simulink model "MicrogridControl"  (R2025b)
settings: Solver=VariableStepAuto  StartTime=0.0  StopTime=8  FixedStep=Ts  RelTol=1e-3
PreLoadFcn:
  | NormalOperation;
  | MicrogridControlParam;
undefined symbols (not defined in the file): base, bessModeInitial, bessSystem, bessVoltage, breakerStatus, DiscIntNeverNeededParam, ee_sli_rtmsupport, event, gcbh, generator, gflInverter, gfmInverter, Inertia, lineInductance, lineResistance, machine, plannedIsland, pmsm, powerLimit, powerQuality, PV, PVInverter, ref, resync, solar, solarInsolationChange, systemFrequency, Ts, windController, windSystem, windTurbine
libraries: nesl_utility x234, ee_lib x174, fl_lib x143, eeGeneralControl x137, simulink x78, eeTransforms x47, slpidlib x23, nesl_utility_internal x12, eePwmGenerator x9, eeSinusoidalMeasurementV2 x9, custom_lib x7, batteryecm_lib x6
(part 5 of 25)

== system MicrogridControl/Subsystem/Subsystem1 ==
  Current and Voltage Sensor (Three-Phase) : ee_lib/Sensors & Transducers/Current and Voltage Sensor (Three-Phase)  vMeasurementType=ee.enum.vmeasurement.ll  outputUnit=ee.enum.unit.si  SRated=100e6 A*V  VRated=24e3 V  I_specify=off  I_priority=None  I=[0, 0, 0] A  I_nominal_specify=off  I_nominal_value=1  I_nominal_unit=A  V_specify=off  V_priority=None  V=[0, 0, 0] V  V_nominal_specify=off  V_nominal_value=1  V_nominal_unit=V
      settings: InternalSimscapePortConfiguration="{\"Bottom\":[],\"Left\":[{\"id\":\"N1\",\"label\":\"~1\",\"type\":\"foundation.electrical.three_phase\"}],\"Right\":[{\"id\":\"V_output\",\"label\":\"V\",\"type\":\"output\"},{\"id\":\"I_output\",\"label\":\"I\",\"type\":\"output\"},{\"id\":\"N2\",\"label\":\"~2\",\"type\":\"foundation.electrical.three_phase\"}],\"Top\":[]}"
  Low-Pass Filter (Discrete or Continuous) : eeGeneralControl/Low-Pass Filter (Discrete or Continuous)  K=1  T=0.1  B=inf  A=-inf  init_option=Inherited from block input  x0=0  Ts=-1
  Low-Pass Filter (Discrete or Continuous)1 : eeGeneralControl/Low-Pass Filter (Discrete or Continuous)  K=1  T=0.1  B=inf  A=-inf  init_option=Inherited from block input  x0=0  Ts=-1
  PS-Simulink Converter : nesl_utility/PS-Simulink Converter  PhysicalDomain=network_engine_domain  SubClassName=ps_output  LeftPortType=input  RightPortType=output  PseudoPeriodic=off  Frequencies=[]  VectorFormat=inherit  Unit=inherit  AffineConversion=off
  PS-Simulink Converter1 : nesl_utility/PS-Simulink Converter  PhysicalDomain=network_engine_domain  SubClassName=ps_output  LeftPortType=input  RightPortType=output  PseudoPeriodic=off  Frequencies=[]  VectorFormat=inherit  Unit=inherit  AffineConversion=off
  PS-Simulink Converter2 : nesl_utility/PS-Simulink Converter  PhysicalDomain=network_engine_domain  SubClassName=ps_output  LeftPortType=input  RightPortType=output  PseudoPeriodic=off  Frequencies=[]  VectorFormat=inherit  Unit=MW  AffineConversion=off
  PS-Simulink Converter3 : nesl_utility/PS-Simulink Converter  PhysicalDomain=network_engine_domain  SubClassName=ps_output  LeftPortType=input  RightPortType=output  PseudoPeriodic=off  Frequencies=[]  VectorFormat=inherit  Unit=MW  AffineConversion=off
  Power Sensor (Three-Phase) : ee_lib/Sensors & Transducers/Power Sensor (Three-Phase)  load_type=ee.enum.passive.type_balanced.balanced  f0=60 Hz
      settings: InternalSimscapePortConfiguration="{\"Bottom\":[],\"Left\":[{\"id\":\"N1\",\"label\":\"~1\",\"type\":\"foundation.electrical.three_phase\"}],\"Right\":[{\"id\":\"N2\",\"label\":\"~2\",\"type\":\"foundation.electrical.three_phase\"}],\"Top\":[{\"id\":\"Pm\",\"label\":\"P\",\"type\":\"output\"},{\"id\":\"Qm\",\"label\":\"Q\",\"type\":\"output\"}]}"
  Scope : Scope  NumInputPorts=2
      settings: ActiveDisplayYMinimum=-13008.240762880825  ActiveDisplayYMaximum=11933.172671563581
  In : PMIOPort  Side=Left
  Out : PMIOPort  Port=2  Side=Right
  Q : Outport
  P : Outport  Port=2
  wires:
  PS-Simulink Converter/1 -> Scope/1
  PS-Simulink Converter1/1 -> Scope/2
  PS-Simulink Converter3/1 -> Low-Pass Filter (Discrete or Continuous)1/1
  PS-Simulink Converter2/1 -> Low-Pass Filter (Discrete or Continuous)/1
  Low-Pass Filter (Discrete or Continuous)/1 -> P/1
  Low-Pass Filter (Discrete or Continuous)1/1 -> Q/1
  connections:
  PS-Simulink Converter/LConn1 -- Current and Voltage Sensor (Three-Phase)/RConn1
  Power Sensor (Three-Phase)/LConn1 -- Current and Voltage Sensor (Three-Phase)/RConn3
  Current and Voltage Sensor (Three-Phase)/LConn1 -- In/RConn1
  Power Sensor (Three-Phase)/RConn1 -- Out/RConn1
  PS-Simulink Converter1/LConn1 -- Current and Voltage Sensor (Three-Phase)/RConn2
  PS-Simulink Converter2/LConn1 -- Power Sensor (Three-Phase)/LConn2
  PS-Simulink Converter3/LConn1 -- Power Sensor (Three-Phase)/LConn3

== system MicrogridControl/Subsystem1/Circuit Breaker ==
  BRK : Inport
  Data Type Conversion : DataTypeConversion  OutDataTypeStr=double  SaturateOnIntegerOverflow=off  RndMeth=Floor
  Open Resistance : Gain  Gain=5e6
  Phase Splitter : ee_lib/Connectors & References/Phase Splitter
  Phase Splitter1 : ee_lib/Connectors & References/Phase Splitter
  Simulink-PS Converter : nesl_utility/Simulink-PS Converter  PhysicalDomain=network_engine_domain  SubClassName=ps_input  LeftPortType=input  RightPortType=output  PseudoPeriodic=off  Frequencies=[]  NoiseDistribution=none  NoiseParameters=[]  Unit=1  AffineConversion=off  FilteringAndDerivatives=provide  SimscapeFilterOrder=1  InputFilterTimeConstant=0.001  UdotUserProvided=0
  Variable Resistor : fl_lib/Electrical/Electrical Elements/Variable Resistor  Rmin=1e-3 Ohm  thermalEnable=false  thermal_mass=1 J/K  i_specify=on  i_priority=None  i=0 A  i_nominal_specify=off  i_nominal_value=1  i_nominal_unit=A  v_specify=off  v_priority=None  v=0 V  v_nominal_specify=off  v_nominal_value=1  v_nominal_unit=V  T_specify=off  T_priority=None  T=300 K  T_nominal_specify=off  T_nominal_value=1  T_nominal_unit=K
  Variable Resistor1 : fl_lib/Electrical/Electrical Elements/Variable Resistor  Rmin=1e-3 Ohm  thermalEnable=false  thermal_mass=1 J/K  i_specify=on  i_priority=None  i=0 A  i_nominal_specify=off  i_nominal_value=1  i_nominal_unit=A  v_specify=off  v_priority=None  v=0 V  v_nominal_specify=off  v_nominal_value=1  v_nominal_unit=V  T_specify=off  T_priority=None  T=300 K  T_nominal_specify=off  T_nominal_value=1  T_nominal_unit=K
  Variable Resistor2 : fl_lib/Electrical/Electrical Elements/Variable Resistor  Rmin=1e-3 Ohm  thermalEnable=false  thermal_mass=1 J/K  i_specify=on  i_priority=None  i=0 A  i_nominal_specify=off  i_nominal_value=1  i_nominal_unit=A  v_specify=off  v_priority=None  v=0 V  v_nominal_specify=off  v_nominal_value=1  v_nominal_unit=V  T_specify=off  T_priority=None  T=300 K  T_nominal_specify=off  T_nominal_value=1  T_nominal_unit=K
  In : PMIOPort  Side=Left
  ~ : PMIOPort  Port=2  Side=Right
  wires:
  Data Type Conversion/1 -> Open Resistance/1
  BRK/1 -> Data Type Conversion/1
  Open Resistance/1 -> Simulink-PS Converter/1
  connections:
  Phase Splitter1/RConn2 -- Variable Resistor1/RConn1
  Variable Resistor1/LConn2 -- Phase Splitter/RConn2
  Phase Splitter1/RConn3 -- Variable Resistor2/RConn1
  Phase Splitter/RConn1 -- Variable Resistor/LConn2
  Variable Resistor2/LConn2 -- Phase Splitter/RConn3
  Phase Splitter1/RConn1 -- Variable Resistor/RConn1
  Phase Splitter1/LConn1 -- ~/RConn1
  Variable Resistor/LConn1 -- Simulink-PS Converter/RConn1 -- Variable Resistor2/LConn1 -- Variable Resistor1/LConn1
  Phase Splitter/LConn1 -- In/RConn1

== system MicrogridControl/Subsystem1/Subsystem9 ==
  Current and Voltage Sensor (Three-Phase) : ee_lib/Sensors & Transducers/Current and Voltage Sensor (Three-Phase)  vMeasurementType=ee.enum.vmeasurement.ll  outputUnit=ee.enum.unit.si  SRated=100e6 A*V  VRated=24e3 V  I_specify=off  I_priority=None  I=[0, 0, 0] A  I_nominal_specify=off  I_nominal_value=1  I_nominal_unit=A  V_specify=off  V_priority=None  V=[0, 0, 0] V  V_nominal_specify=off  V_nominal_value=1  V_nominal_unit=V
      settings: InternalSimscapePortConfiguration="{\"Bottom\":[],\"Left\":[{\"id\":\"N1\",\"label\":\"~1\",\"type\":\"foundation.electrical.three_phase\"}],\"Right\":[{\"id\":\"V_output\",\"label\":\"V\",\"type\":\"output\"},{\"id\":\"I_output\",\"label\":\"I\",\"type\":\"output\"},{\"id\":\"N2\",\"label\":\"~2\",\"type\":\"foundation.electrical.three_phase\"}],\"Top\":[]}"
  Low-Pass Filter (Discrete or Continuous) : eeGeneralControl/Low-Pass Filter (Discrete or Continuous)  K=1  T=0.1  B=inf  A=-inf  init_option=Inherited from block input  x0=0  Ts=-1
  PS-Simulink Converter : nesl_utility/PS-Simulink Converter  PhysicalDomain=network_engine_domain  SubClassName=ps_output  LeftPortType=input  RightPortType=output  PseudoPeriodic=off  Frequencies=[]  VectorFormat=inherit  Unit=inherit  AffineConversion=off
  PS-Simulink Converter1 : nesl_utility/PS-Simulink Converter  PhysicalDomain=network_engine_domain  SubClassName=ps_output  LeftPortType=input  RightPortType=output  PseudoPeriodic=off  Frequencies=[]  VectorFormat=inherit  Unit=inherit  AffineConversion=off
  PS-Simulink Converter2 : nesl_utility/PS-Simulink Converter  PhysicalDomain=network_engine_domain  SubClassName=ps_output  LeftPortType=input  RightPortType=output  PseudoPeriodic=off  Frequencies=[]  VectorFormat=inherit  Unit=MW  AffineConversion=off
  PS-Simulink Converter3 : nesl_utility/PS-Simulink Converter  PhysicalDomain=network_engine_domain  SubClassName=ps_output  LeftPortType=input  RightPortType=output  PseudoPeriodic=off  Frequencies=[]  VectorFormat=inherit  Unit=MW  AffineConversion=off
  Power Sensor (Three-Phase) : ee_lib/Sensors & Transducers/Power Sensor (Three-Phase)  load_type=ee.enum.passive.type_balanced.balanced  f0=60 Hz
      settings: InternalSimscapePortConfiguration="{\"Bottom\":[],\"Left\":[{\"id\":\"N1\",\"label\":\"~1\",\"type\":\"foundation.electrical.three_phase\"}],\"Right\":[{\"id\":\"N2\",\"label\":\"~2\",\"type\":\"foundation.electrical.three_phase\"}],\"Top\":[{\"id\":\"Pm\",\"label\":\"P\",\"type\":\"output\"},{\"id\":\"Qm\",\"label\":\"Q\",\"type\":\"output\"}]}"
  Scope : Scope  NumInputPorts=2
      settings: ActiveDisplayYMinimum=-149653.61636  ActiveDisplayYMaximum=88760.25757
  Scope1 : Scope  NumInputPorts=2
      settings: ActiveDisplayYMinimum=-1.31777056807E+6  ActiveDisplayYMaximum=1.0009721031E+6  DataLoggingVariableName=ScopeData2
  In : PMIOPort  Side=Left
  Out : PMIOPort  Port=2  Side=Right
  Q : Outport
  P : Outport  Port=2
  wires:
  PS-Simulink Converter/1 -> Scope/1
  PS-Simulink Converter1/1 -> Scope/2
  PS-Simulink Converter3/1 -> Q/1, Scope1/2
  PS-Simulink Converter2/1 -> Low-Pass Filter (Discrete or Continuous)/1, Scope1/1
  Low-Pass Filter (Discrete or Continuous)/1 -> P/1
  connections:
  PS-Simulink Converter/LConn1 -- Current and Voltage Sensor (Three-Phase)/RConn1
  Power Sensor (Three-Phase)/LConn1 -- Current and Voltage Sensor (Three-Phase)/RConn3
  Current and Voltage Sensor (Three-Phase)/LConn1 -- In/RConn1
  Power Sensor (Three-Phase)/RConn1 -- Out/RConn1
  PS-Simulink Converter1/LConn1 -- Current and Voltage Sensor (Three-Phase)/RConn2
  PS-Simulink Converter2/LConn1 -- Power Sensor (Three-Phase)/LConn2
  PS-Simulink Converter3/LConn1 -- Power Sensor (Three-Phase)/LConn3

== system MicrogridControl/Subsystem13/Subsystem ==
  Current and Voltage Sensor (Three-Phase) : ee_lib/Sensors & Transducers/Current and Voltage Sensor (Three-Phase)  vMeasurementType=ee.enum.vmeasurement.ll  outputUnit=ee.enum.unit.si  SRated=100e6 A*V  VRated=24e3 V  I_specify=off  I_priority=None  I=[0, 0, 0] A  I_nominal_specify=off  I_nominal_value=1  I_nominal_unit=A  V_specify=off  V_priority=None  V=[0, 0, 0] V  V_nominal_specify=off  V_nominal_value=1  V_nominal_unit=V
      settings: InternalSimscapePortConfiguration="{\"Bottom\":[],\"Left\":[{\"id\":\"N1\",\"label\":\"~1\",\"type\":\"foundation.electrical.three_phase\"}],\"Right\":[{\"id\":\"V_output\",\"label\":\"V\",\"type\":\"output\"},{\"id\":\"I_output\",\"label\":\"I\",\"type\":\"output\"},{\"id\":\"N2\",\"label\":\"~2\",\"type\":\"foundation.electrical.three_phase\"}],\"Top\":[]}"
  Low-Pass Filter (Discrete or Continuous) : eeGeneralControl/Low-Pass Filter (Discrete or Continuous)  K=1  T=0.1  B=inf  A=-inf  init_option=Inherited from block input  x0=0  Ts=-1
  Low-Pass Filter (Discrete or Continuous)1 : eeGeneralControl/Low-Pass Filter (Discrete or Continuous)  K=1  T=0.1  B=inf  A=-inf  init_option=Inherited from block input  x0=0  Ts=-1
  PS-Simulink Converter : nesl_utility/PS-Simulink Converter  PhysicalDomain=network_engine_domain  SubClassName=ps_output  LeftPortType=input  RightPortType=output  PseudoPeriodic=off  Frequencies=[]  VectorFormat=inherit  Unit=inherit  AffineConversion=off
  PS-Simulink Converter1 : nesl_utility/PS-Simulink Converter  PhysicalDomain=network_engine_domain  SubClassName=ps_output  LeftPortType=input  RightPortType=output  PseudoPeriodic=off  Frequencies=[]  VectorFormat=inherit  Unit=inherit  AffineConversion=off
  PS-Simulink Converter2 : nesl_utility/PS-Simulink Converter  PhysicalDomain=network_engine_domain  SubClassName=ps_output  LeftPortType=input  RightPortType=output  PseudoPeriodic=off  Frequencies=[]  VectorFormat=inherit  Unit=MW  AffineConversion=off
  PS-Simulink Converter3 : nesl_utility/PS-Simulink Converter  PhysicalDomain=network_engine_domain  SubClassName=ps_output  LeftPortType=input  RightPortType=output  PseudoPeriodic=off  Frequencies=[]  VectorFormat=inherit  Unit=MW  AffineConversion=off
  Power Sensor (Three-Phase) : ee_lib/Sensors & Transducers/Power Sensor (Three-Phase)  load_type=ee.enum.passive.type_balanced.balanced  f0=60 Hz
      settings: InternalSimscapePortConfiguration="{\"Bottom\":[],\"Left\":[{\"id\":\"N1\",\"label\":\"~1\",\"type\":\"foundation.electrical.three_phase\"}],\"Right\":[{\"id\":\"N2\",\"label\":\"~2\",\"type\":\"foundation.electrical.three_phase\"}],\"Top\":[{\"id\":\"Pm\",\"label\":\"P\",\"type\":\"output\"},{\"id\":\"Qm\",\"label\":\"Q\",\"type\":\"output\"}]}"
  Scope : Scope  NumInputPorts=2
      settings: ActiveDisplayYMinimum=-149653.61636  ActiveDisplayYMaximum=88760.25757
  In : PMIOPort  Side=Left
  Out : PMIOPort  Port=2  Side=Right
  Q : Outport
  P : Outport  Port=2
  wires:
  PS-Simulink Converter/1 -> Scope/1
  PS-Simulink Converter1/1 -> Scope/2
  PS-Simulink Converter3/1 -> Low-Pass Filter (Discrete or Continuous)1/1
  PS-Simulink Converter2/1 -> Low-Pass Filter (Discrete or Continuous)/1
  Low-Pass Filter (Discrete or Continuous)/1 -> P/1
  Low-Pass Filter (Discrete or Continuous)1/1 -> Q/1
  connections:
  PS-Simulink Converter/LConn1 -- Current and Voltage Sensor (Three-Phase)/RConn1
  Power Sensor (Three-Phase)/LConn1 -- Current and Voltage Sensor (Three-Phase)/RConn3
  Current and Voltage Sensor (Three-Phase)/LConn1 -- In/RConn1
  Power Sensor (Three-Phase)/RConn1 -- Out/RConn1
  PS-Simulink Converter1/LConn1 -- Current and Voltage Sensor (Three-Phase)/RConn2
  PS-Simulink Converter2/LConn1 -- Power Sensor (Three-Phase)/LConn2
  PS-Simulink Converter3/LConn1 -- Power Sensor (Three-Phase)/LConn3

== system MicrogridControl/Subsystem15/Circuit Breaker ==
  BRK : Inport
  Data Type Conversion : DataTypeConversion  OutDataTypeStr=double  SaturateOnIntegerOverflow=off  RndMeth=Floor
  Open Resistance : Gain  Gain=5e6
  Phase Splitter : ee_lib/Connectors & References/Phase Splitter
  Phase Splitter1 : ee_lib/Connectors & References/Phase Splitter
  Simulink-PS Converter : nesl_utility/Simulink-PS Converter  PhysicalDomain=network_engine_domain  SubClassName=ps_input  LeftPortType=input  RightPortType=output  PseudoPeriodic=off  Frequencies=[]  NoiseDistribution=none  NoiseParameters=[]  Unit=1  AffineConversion=off  FilteringAndDerivatives=provide  SimscapeFilterOrder=1  InputFilterTimeConstant=0.001  UdotUserProvided=0
  Variable Resistor : fl_lib/Electrical/Electrical Elements/Variable Resistor  Rmin=1e-3 Ohm  thermalEnable=false  thermal_mass=1 J/K  i_specify=on  i_priority=None  i=0 A  i_nominal_specify=off  i_nominal_value=1  i_nominal_unit=A  v_specify=off  v_priority=None  v=0 V  v_nominal_specify=off  v_nominal_value=1  v_nominal_unit=V  T_specify=off  T_priority=None  T=300 K  T_nominal_specify=off  T_nominal_value=1  T_nominal_unit=K
  Variable Resistor1 : fl_lib/Electrical/Electrical Elements/Variable Resistor  Rmin=1e-3 Ohm  thermalEnable=false  thermal_mass=1 J/K  i_specify=on  i_priority=None  i=0 A  i_nominal_specify=off  i_nominal_value=1  i_nominal_unit=A  v_specify=off  v_priority=None  v=0 V  v_nominal_specify=off  v_nominal_value=1  v_nominal_unit=V  T_specify=off  T_priority=None  T=300 K  T_nominal_specify=off  T_nominal_value=1  T_nominal_unit=K
  Variable Resistor2 : fl_lib/Electrical/Electrical Elements/Variable Resistor  Rmin=1e-3 Ohm  thermalEnable=false  thermal_mass=1 J/K  i_specify=on  i_priority=None  i=0 A  i_nominal_specify=off  i_nominal_value=1  i_nominal_unit=A  v_specify=off  v_priority=None  v=0 V  v_nominal_specify=off  v_nominal_value=1  v_nominal_unit=V  T_specify=off  T_priority=None  T=300 K  T_nominal_specify=off  T_nominal_value=1  T_nominal_unit=K
  In : PMIOPort  Side=Left
  ~ : PMIOPort  Port=2  Side=Right
  wires:
  Data Type Conversion/1 -> Open Resistance/1
  BRK/1 -> Data Type Conversion/1
  Open Resistance/1 -> Simulink-PS Converter/1
  connections:
  Phase Splitter1/RConn2 -- Variable Resistor1/RConn1
  Variable Resistor1/LConn2 -- Phase Splitter/RConn2
  Phase Splitter1/RConn3 -- Variable Resistor2/RConn1
  Phase Splitter/RConn1 -- Variable Resistor/LConn2
  Variable Resistor2/LConn2 -- Phase Splitter/RConn3
  Phase Splitter1/RConn1 -- Variable Resistor/RConn1
  Phase Splitter1/LConn1 -- ~/RConn1
  Variable Resistor/LConn1 -- Simulink-PS Converter/RConn1 -- Variable Resistor2/LConn1 -- Variable Resistor1/LConn1
  Phase Splitter/LConn1 -- In/RConn1

== system MicrogridControl/Subsystem15/Subsystem4 ==
  Current and Voltage Sensor (Three-Phase) : ee_lib/Sensors & Transducers/Current and Voltage Sensor (Three-Phase)  vMeasurementType=ee.enum.vmeasurement.ll  outputUnit=ee.enum.unit.si  SRated=100e6 A*V  VRated=24e3 V  I_specify=off  I_priority=None  I=[0, 0, 0] A  I_nominal_specify=off  I_nominal_value=1  I_nominal_unit=A  V_specify=off  V_priority=None  V=[0, 0, 0] V  V_nominal_specify=off  V_nominal_value=1  V_nominal_unit=V
      settings: InternalSimscapePortConfiguration="{\"Bottom\":[],\"Left\":[{\"id\":\"N1\",\"label\":\"~1\",\"type\":\"foundation.electrical.three_phase\"}],\"Right\":[{\"id\":\"V_output\",\"label\":\"V\",\"type\":\"output\"},{\"id\":\"I_output\",\"label\":\"I\",\"type\":\"output\"},{\"id\":\"N2\",\"label\":\"~2\",\"type\":\"foundation.electrical.three_phase\"}],\"Top\":[]}"
  Gain : Gain  Gain=0.5
  Low-Pass Filter (Discrete or Continuous) : eeGeneralControl/Low-Pass Filter (Discrete or Continuous)  K=1  T=0.1  B=inf  A=-inf  init_option=Inherited from block input  x0=0  Ts=-1
  Low-Pass Filter (Discrete or Continuous)1 : eeGeneralControl/Low-Pass Filter (Discrete or Continuous)  K=1  T=0.1  B=inf  A=-inf  init_option=Inherited from block input  x0=0  Ts=-1
  PS-Simulink Converter : nesl_utility/PS-Simulink Converter  PhysicalDomain=network_engine_domain  SubClassName=ps_output  LeftPortType=input  RightPortType=output  PseudoPeriodic=off  Frequencies=[]  VectorFormat=inherit  Unit=inherit  AffineConversion=off
  PS-Simulink Converter1 : nesl_utility/PS-Simulink Converter  PhysicalDomain=network_engine_domain  SubClassName=ps_output  LeftPortType=input  RightPortType=output  PseudoPeriodic=off  Frequencies=[]  VectorFormat=inherit  Unit=inherit  AffineConversion=off
  PS-Simulink Converter2 : nesl_utility/PS-Simulink Converter  PhysicalDomain=network_engine_domain  SubClassName=ps_output  LeftPortType=input  RightPortType=output  PseudoPeriodic=off  Frequencies=[]  VectorFormat=inherit  Unit=MW  AffineConversion=off
  PS-Simulink Converter3 : nesl_utility/PS-Simulink Converter  PhysicalDomain=network_engine_domain  SubClassName=ps_output  LeftPortType=input  RightPortType=output  PseudoPeriodic=off  Frequencies=[]  VectorFormat=inherit  Unit=MW  AffineConversion=off
  Power Sensor (Three-Phase) : ee_lib/Sensors & Transducers/Power Sensor (Three-Phase)  load_type=ee.enum.passive.type_balanced.balanced  f0=60 Hz
      settings: InternalSimscapePortConfiguration="{\"Bottom\":[],\"Left\":[{\"id\":\"N1\",\"label\":\"~1\",\"type\":\"foundation.electrical.three_phase\"}],\"Right\":[{\"id\":\"N2\",\"label\":\"~2\",\"type\":\"foundation.electrical.three_phase\"}],\"Top\":[{\"id\":\"Pm\",\"label\":\"P\",\"type\":\"output\"},{\"id\":\"Qm\",\"label\":\"Q\",\"type\":\"output\"}]}"
  Scope : Scope  NumInputPorts=2
      settings: ActiveDisplayYMinimum=-149653.61636  ActiveDisplayYMaximum=88760.25757
  In : PMIOPort  Side=Left
  Out : PMIOPort  Port=2  Side=Right
  Q : Outport
  P : Outport  Port=2
  wires:
  PS-Simulink Converter/1 -> Scope/1
  PS-Simulink Converter1/1 -> Scope/2
  PS-Simulink Converter2/1 -> Low-Pass Filter (Discrete or Continuous)/1
  Low-Pass Filter (Discrete or Continuous)/1 -> P/1
  PS-Simulink Converter3/1 -> Low-Pass Filter (Discrete or Continuous)1/1
  Low-Pass Filter (Discrete or Continuous)1/1 -> Q/1
  connections:
  PS-Simulink Converter/LConn1 -- Current and Voltage Sensor (Three-Phase)/RConn1
  Power Sensor (Three-Phase)/LConn1 -- Current and Voltage Sensor (Three-Phase)/RConn3
  Current and Voltage Sensor (Three-Phase)/LConn1 -- In/RConn1
  Power Sensor (Three-Phase)/RConn1 -- Out/RConn1
  PS-Simulink Converter1/LConn1 -- Current and Voltage Sensor (Three-Phase)/RConn2
  PS-Simulink Converter2/LConn1 -- Power Sensor (Three-Phase)/LConn2
  PS-Simulink Converter3/LConn1 -- Power Sensor (Three-Phase)/LConn3

== system MicrogridControl/Subsystem15/Transformer ==
  Detailed : Subsystem  VariantControl=Detailed
  Simplified : Subsystem  VariantControl=Simplified  mask{windingRatio=13500/6600}
      mask prompts: windingRatio "Winding ratio"
      mask DialogControl Container4 Prompt: General
  In : PMIOPort  Side=Left
  Out : PMIOPort  Port=2  Side=Right

== system MicrogridControl/Subsystem3/Subsystem2 ==
  Current and Voltage Sensor (Three-Phase) : ee_lib/Sensors & Transducers/Current and Voltage Sensor (Three-Phase)  vMeasurementType=ee.enum.vmeasurement.ll  outputUnit=ee.enum.unit.pu  SRated=10.5e6 A*V  VRated=11000 V  I_specify=off  I_priority=None  I=[0, 0, 0] A  I_nominal_specify=off  I_nominal_value=1  I_nominal_unit=A  V_specify=off  V_priority=None  V=[0, 0, 0] V  V_nominal_specify=off  V_nominal_value=1  V_nominal_unit=V
      settings: InternalSimscapePortConfiguration="{\"Bottom\":[],\"Left\":[{\"id\":\"N1\",\"label\":\"~1\",\"type\":\"foundation.electrical.three_phase\"}],\"Right\":[{\"id\":\"V_output\",\"label\":\"V\",\"type\":\"output\"},{\"id\":\"I_output\",\"label\":\"I\",\"type\":\"output\"},{\"id\":\"N2\",\"label\":\"~2\",\"type\":\"foundation.electrical.three_phase\"}],\"Top\":[]}"
  Low-Pass Filter (Discrete or Continuous) : eeGeneralControl/Low-Pass Filter (Discrete or Continuous)  K=1  T=0.1  B=inf  A=-inf  init_option=Inherited from block input  x0=0  Ts=-1
  Low-Pass Filter (Discrete or Continuous)1 : eeGeneralControl/Low-Pass Filter (Discrete or Continuous)  K=1  T=0.1  B=inf  A=-inf  init_option=Inherited from block input  x0=0  Ts=-1
  Low-Pass Filter (Discrete or Continuous)2 : eeGeneralControl/Low-Pass Filter (Discrete or Continuous)  K=1  T=0.001  B=inf  A=-inf  init_option=Inherited from block input  x0=0  Ts=-1
  Low-Pass Filter (Discrete or Continuous)3 : eeGeneralControl/Low-Pass Filter (Discrete or Continuous)  K=1  T=0.001  B=inf  A=-inf  init_option=Inherited from block input  x0=0  Ts=-1
  PS-Simulink Converter : nesl_utility/PS-Simulink Converter  PhysicalDomain=network_engine_domain  SubClassName=ps_output  LeftPortType=input  RightPortType=output  PseudoPeriodic=off  Frequencies=[]  VectorFormat=inherit  Unit=inherit  AffineConversion=off
  PS-Simulink Converter1 : nesl_utility/PS-Simulink Converter  PhysicalDomain=network_engine_domain  SubClassName=ps_output  LeftPortType=input  RightPortType=output  PseudoPeriodic=off  Frequencies=[]  VectorFormat=inherit  Unit=inherit  AffineConversion=off
  PS-Simulink Converter2 : nesl_utility/PS-Simulink Converter  PhysicalDomain=network_engine_domain  SubClassName=ps_output  LeftPortType=input  RightPortType=output  PseudoPeriodic=off  Frequencies=[]  VectorFormat=inherit  Unit=MW  AffineConversion=off
  PS-Simulink Converter3 : nesl_utility/PS-Simulink Converter  PhysicalDomain=network_engine_domain  SubClassName=ps_output  LeftPortType=input  RightPortType=output  PseudoPeriodic=off  Frequencies=[]  VectorFormat=inherit  Unit=MW  AffineConversion=off
  Power Sensor (Three-Phase) : ee_lib/Sensors & Transducers/Power Sensor (Three-Phase)  load_type=ee.enum.passive.type_balanced.balanced  f0=60 Hz
      settings: InternalSimscapePortConfiguration="{\"Bottom\":[],\"Left\":[{\"id\":\"N1\",\"label\":\"~1\",\"type\":\"foundation.electrical.three_phase\"}],\"Right\":[{\"id\":\"N2\",\"label\":\"~2\",\"type\":\"foundation.electrical.three_phase\"}],\"Top\":[{\"id\":\"Pm\",\"label\":\"P\",\"type\":\"output\"},{\"id\":\"Qm\",\"label\":\"Q\",\"type\":\"output\"}]}"
  Terminator : Terminator
  Terminator1 : Terminator
  In : PMIOPort  Side=Left
  Out : PMIOPort  Port=2  Side=Right
  P : Outport
  Q : Outport  Port=2
  wires:
  PS-Simulink Converter3/1 -> Low-Pass Filter (Discrete or Continuous)1/1
  PS-Simulink Converter2/1 -> Low-Pass Filter (Discrete or Continuous)/1
  Low-Pass Filter (Discrete or Continuous)/1 -> P/1
  Low-Pass Filter (Discrete or Continuous)1/1 -> Q/1
  PS-Simulink Converter/1 -> Low-Pass Filter (Discrete or Continuous)2/1
  Low-Pass Filter (Discrete or Continuous)2/1 -> Terminator/1
  PS-Simulink Converter1/1 -> Low-Pass Filter (Discrete or Continuous)3/1
  Low-Pass Filter (Discrete or Continuous)3/1 -> Terminator1/1
  connections:
  PS-Simulink Converter/LConn1 -- Current and Voltage Sensor (Three-Phase)/RConn1
  Power Sensor (Three-Phase)/LConn1 -- Current and Voltage Sensor (Three-Phase)/RConn3
  Current and Voltage Sensor (Three-Phase)/LConn1 -- In/RConn1
  Power Sensor (Three-Phase)/RConn1 -- Out/RConn1
  PS-Simulink Converter1/LConn1 -- Current and Voltage Sensor (Three-Phase)/RConn2
  PS-Simulink Converter2/LConn1 -- Power Sensor (Three-Phase)/LConn2
  PS-Simulink Converter3/LConn1 -- Power Sensor (Three-Phase)/LConn3

== system MicrogridControl/Subsystem4/Subsystem3 ==
  Current and Voltage Sensor (Three-Phase) : ee_lib/Sensors & Transducers/Current and Voltage Sensor (Three-Phase)  vMeasurementType=ee.enum.vmeasurement.ll  outputUnit=ee.enum.unit.si  SRated=100e6 A*V  VRated=24e3 V  I_specify=off  I_priority=None  I=[0, 0, 0] A  I_nominal_specify=off  I_nominal_value=1  I_nominal_unit=A  V_specify=off  V_priority=None  V=[0, 0, 0] V  V_nominal_specify=off  V_nominal_value=1  V_nominal_unit=V
      settings: InternalSimscapePortConfiguration="{\"Bottom\":[],\"Left\":[{\"id\":\"N1\",\"label\":\"~1\",\"type\":\"foundation.electrical.three_phase\"}],\"Right\":[{\"id\":\"V_output\",\"label\":\"V\",\"type\":\"output\"},{\"id\":\"I_output\",\"label\":\"I\",\"type\":\"output\"},{\"id\":\"N2\",\"label\":\"~2\",\"type\":\"foundation.electrical.three_phase\"}],\"Top\":[]}"
  Low-Pass Filter (Discrete or Continuous) : eeGeneralControl/Low-Pass Filter (Discrete or Continuous)  K=1  T=0.1  B=inf  A=-inf  init_option=Inherited from block input  x0=0  Ts=-1
  Low-Pass Filter (Discrete or Continuous)1 : eeGeneralControl/Low-Pass Filter (Discrete or Continuous)  K=1  T=0.1  B=inf  A=-inf  init_option=Inherited from block input  x0=0  Ts=-1
  PS-Simulink Converter : nesl_utility/PS-Simulink Converter  PhysicalDomain=network_engine_domain  SubClassName=ps_output  LeftPortType=input  RightPortType=output  PseudoPeriodic=off  Frequencies=[]  VectorFormat=inherit  Unit=inherit  AffineConversion=off
  PS-Simulink Converter1 : nesl_utility/PS-Simulink Converter  PhysicalDomain=network_engine_domain  SubClassName=ps_output  LeftPortType=input  RightPortType=output  PseudoPeriodic=off  Frequencies=[]  VectorFormat=inherit  Unit=inherit  AffineConversion=off
  PS-Simulink Converter2 : nesl_utility/PS-Simulink Converter  PhysicalDomain=network_engine_domain  SubClassName=ps_output  LeftPortType=input  RightPortType=output  PseudoPeriodic=off  Frequencies=[]  VectorFormat=inherit  Unit=MW  AffineConversion=off
  PS-Simulink Converter3 : nesl_utility/PS-Simulink Converter  PhysicalDomain=network_engine_domain  SubClassName=ps_output  LeftPortType=input  RightPortType=output  PseudoPeriodic=off  Frequencies=[]  VectorFormat=inherit  Unit=MW  AffineConversion=off
  Power Sensor (Three-Phase) : ee_lib/Sensors & Transducers/Power Sensor (Three-Phase)  load_type=ee.enum.passive.type_balanced.balanced  f0=60 Hz
      settings: InternalSimscapePortConfiguration="{\"Bottom\":[],\"Left\":[{\"id\":\"N1\",\"label\":\"~1\",\"type\":\"foundation.electrical.three_phase\"}],\"Right\":[{\"id\":\"N2\",\"label\":\"~2\",\"type\":\"foundation.electrical.three_phase\"}],\"Top\":[{\"id\":\"Pm\",\"label\":\"P\",\"type\":\"output\"},{\"id\":\"Qm\",\"label\":\"Q\",\"type\":\"output\"}]}"
  Scope : Scope  NumInputPorts=2
      settings: ActiveDisplayYMinimum=-149653.61636  ActiveDisplayYMaximum=88760.25757
  In : PMIOPort  Side=Left
  Out : PMIOPort  Port=2  Side=Right
  Q : Outport
  P : Outport  Port=2
  wires:
  PS-Simulink Converter/1 -> Scope/1
  PS-Simulink Converter1/1 -> Scope/2
  PS-Simulink Converter3/1 -> Low-Pass Filter (Discrete or Continuous)1/1
  PS-Simulink Converter2/1 -> Low-Pass Filter (Discrete or Continuous)/1
  Low-Pass Filter (Discrete or Continuous)/1 -> P/1
  Low-Pass Filter (Discrete or Continuous)1/1 -> Q/1
  connections:
  PS-Simulink Converter/LConn1 -- Current and Voltage Sensor (Three-Phase)/RConn1
  Power Sensor (Three-Phase)/LConn1 -- Current and Voltage Sensor (Three-Phase)/RConn3
  Current and Voltage Sensor (Three-Phase)/LConn1 -- In/RConn1
  Power Sensor (Three-Phase)/RConn1 -- Out/RConn1
  PS-Simulink Converter1/LConn1 -- Current and Voltage Sensor (Three-Phase)/RConn2
  PS-Simulink Converter2/LConn1 -- Power Sensor (Three-Phase)/LConn2
  PS-Simulink Converter3/LConn1 -- Power Sensor (Three-Phase)/LConn3

== system MicrogridControl/Wind Farm/Transformer ==
  Detailed : Subsystem  VariantControl=Detailed
  Simplified : Subsystem  VariantControl=Simplified  mask{windingRatio=690/6600}
      mask prompts: windingRatio "Winding ratio"
      mask DialogControl Container4 Prompt: General
  In : PMIOPort  Side=Left
  Out : PMIOPort  Port=2  Side=Right

== system MicrogridControl/Wind Farm/Transformer1 ==
  Detailed : Subsystem  VariantControl=Detailed
  Simplified : Subsystem  VariantControl=Simplified  mask{windingRatio=690/6600}
      mask prompts: windingRatio "Winding ratio"
      mask DialogControl Container4 Prompt: General
  In : PMIOPort  Side=Left
  Out : PMIOPort  Port=2  Side=Right

== system MicrogridControl/Wind Farm/Wind Plant Integrated ==
  LVRT : Inport
  QRef : Inport  Port=2
  WindSpeed : Inport  Port=3
  Detailed : Subsystem  VariantControl=Detailed
      settings: CopyFcn=set_param(gcbh,'LinkStatus','none');
  Simplified : Subsystem  VariantControl=Simplified
  ~ : PMIOPort  Side=Right
  Meas : Outport

== system MicrogridControl/Wind Farm/Wind Plant Integrated1 ==
  LVRT : Inport
  QRef : Inport  Port=2
  WindSpeed : Inport  Port=3
  Detailed : Subsystem  VariantControl=Detailed
      settings: CopyFcn=set_param(gcbh,'LinkStatus','none');
  Simplified : Subsystem  VariantControl=Simplified
  ~ : PMIOPort  Side=Right
  Meas : Outport

== system MicrogridControl/BESS/BESS Integrated/Detailed ==
  note: Plant
  note: Controller
  VRef : Inport
  FRef : Inport  Port=2
  PRef : Inport  Port=3
  QRef : Inport  Port=4
  Mode : Inport  Port=5
  Reset : Inport  Port=6
  BESS Controller : Subsystem  Variant=on  VariantControlMode=label  LabelModeActiveChoice=Grid Forming
  BESS Plant : Subsystem  mask(BESS Plant){converterFidelity=Average, fSw=fSw, ratedVoltage=Vac}
      mask prompts: converterFidelity "Converter Fidelity"; fSw "Switching Frequency (kHz)"; ratedVoltage "Rated voltage on AC side (V)"
      mask help: This block represents the physical interface between the battery and the power converter. It models the electrical and dynamic characteristics of the battery system connected to a converter, while expecting an external control signal for operation
      settings: CopyFcn=set_param(gcbh,'LinkStatus','none');
      mask TypeOptions converterFidelity: Converter/converterFidelity
      mask Callback converterFidelity: component.mask.converterFidelityPlant;
      mask TypeOptions fSw: Converter/fSw
      mask DialogControl Container4 Prompt: General
      mask DialogControl editBattery Prompt: Edit battery parameters
      mask DialogControl editBattery Callback:
      | blockPath = [gcb,'/','Battery'];
      | component.mask.openBlock(blockPath);
      mask DialogControl editConverter Prompt: Edit converter parameters
      mask DialogControl editConverter Callback:
      | converterFidelity = get_param(gcb,'converterFidelity');
      | blockPath = [gcb,'/','Converter','/',converterFidelity,'/','Converter'];
      | component.mask.openBlock(blockPath);
      mask Display: image('battery.png');
  Filter & Measurements : Subsystem
  ~ : PMIOPort  Side=Right
  Meas : Outport
  wires:
  BESS Plant/1(SOC) -> Filter & Measurements/1(SOC)
  FRef/1 -> BESS Controller/2(FRef)
  Mode/1 -> BESS Controller/5(Mode)
  PRef/1 -> BESS Controller/3(PRef)
  Filter & Measurements/1(VIBus) -> BESS Controller/7(VIBus)
  QRef/1 -> BESS Controller/4(QRef)
  VRef/1 -> BESS Controller/1(VRef)
  Reset/1 -> BESS Controller/6(Reset)
  Filter & Measurements/2(Meas) -> Meas/1
  BESS Controller/1(mabc) -> BESS Plant/1(mabc)
  connections:
  Filter & Measurements/RConn1 -- ~/RConn1
  BESS Plant/RConn1 -- Filter & Measurements/LConn1

== system MicrogridControl/BESS/BESS Integrated/Simplified ==
  VRef : Inport
  FRef : Inport  Port=2
  PRef : Inport  Port=3
  QRef : Inport  Port=4
  Mode : Inport  Port=5
  Reset : Inport  Port=6
  Grid Following : Subsystem  VariantControl=Grid Following  mask(BESS GFL Simplified){plantRating=plantRating, Vac=Vac, frequency=frequency, iMaxPU=iMaxPU, efficiency=efficiency, bessVoltage=baseVoltageDC, maxSOC=maxSOC, minSOC=minSOC}
      mask prompts: plantRating "BESS Rating (kW)"; Vac "Rated AC side voltage (phase-phase RMS) (V)"; frequency "Rated electrical frequency at AC side (Hz)"; iMaxPU "Maximum converter current (pu)"; efficiency "Converter Efficiency (%)"; bessVoltage "Nominal BESS voltage (V)"; maxSOC "Maximum operating SOC"; minSOC "Minimum operating SOC"
      mask help: This block models a BESS that synchronizes with grid voltage and frequency using simplified control representation. This block is designed for computational efficiency, ideal for system-level studies in strong grid conditions where detailed transient behavior is less critical.
      settings: CopyFcn=set_param(gcbh,'LinkStatus','none');
      mask DialogControl generalDetailed Prompt: General
      mask DialogControl Container5 Prompt: Battery
      mask DialogControl editBattery Prompt: Edit battery parameters
      mask DialogControl editBattery Callback:
      | blockPath = [gcb,'/','Battery'] ;
      | component.mask.openBlock(blockPath);
  Grid Forming : Subsystem  VariantControl=Grid Forming  mask(BESS GFM Simplified){plantRating=plantRating, Vac=Vac, frequency=frequency, Vdc=baseVoltageDC, iMaxPU=iMaxPU, efficiency=efficiency, activeDroop=activeDroop, reactiveDroop=reactiveDroop, initialSOC=initialSOC, maxSOC=0.95, minSOC=0.1, capacityType=Infinite, capacity=capacity}
      mask prompts: plantRating "BESS Rating (kW)"; Vac "Rated AC side voltage (phase-phase RMS) (V)"; frequency "Rated electrical frequency at AC side (Hz)"; Vdc "Nominal DC bus voltage (V)"; iMaxPU "Maximum converter current (pu)"; efficiency "Converter Efficiency (%)"; activeDroop "Active droop"; reactiveDroop "Reactive droop"; initialSOC "Initial SOC"; maxSOC "Maximum operating SOC"; minSOC "Minimum operating SOC"; capacityType "Battery charge capacity"; capacity "Battery capacity (Ah)"
      mask help: This block models a BESS with generating voltage and frequency reference capabilities. It is optimized for faster simulations while maintaining essential grid-forming behavior, making it suitable for large-scale stability studies or planning scenarios where detailed converter dynamics are not required.
      settings: CopyFcn=set_param(gcbh,'LinkStatus','none');
      mask TypeOptions capacityType: Fixed | Infinite
      mask Callback capacityType: component.mask.configureBatteryCapacity;
      mask DialogControl generalDetailed Prompt: General
      mask DialogControl Container5 Prompt: Battery
  ~ : PMIOPort  Side=Right
  Meas : Outport

== system MicrogridControl/BESS/BESS Integrated1/Detailed ==
  note: Plant
  note: Controller
  VRef : Inport
  FRef : Inport  Port=2
  PRef : Inport  Port=3
  QRef : Inport  Port=4
  Mode : Inport  Port=5
  Reset : Inport  Port=6
  BESS Controller : Subsystem  Variant=on  VariantControlMode=label  LabelModeActiveChoice=Grid Forming
  BESS Plant : Subsystem  mask(BESS Plant){converterFidelity=Average, fSw=fSw, ratedVoltage=Vac}
      mask prompts: converterFidelity "Converter Fidelity"; fSw "Switching Frequency (kHz)"; ratedVoltage "Rated voltage on AC side (V)"
      mask help: This block represents the physical interface between the battery and the power converter. It models the electrical and dynamic characteristics of the battery system connected to a converter, while expecting an external control signal for operation
      settings: CopyFcn=set_param(gcbh,'LinkStatus','none');
      mask TypeOptions converterFidelity: Converter/converterFidelity
      mask Callback converterFidelity: component.mask.converterFidelityPlant;
      mask TypeOptions fSw: Converter/fSw
      mask DialogControl Container4 Prompt: General
      mask DialogControl editBattery Prompt: Edit battery parameters
      mask DialogControl editBattery Callback:
      | blockPath = [gcb,'/','Battery'];
      | component.mask.openBlock(blockPath);
      mask DialogControl editConverter Prompt: Edit converter parameters
      mask DialogControl editConverter Callback:
      | converterFidelity = get_param(gcb,'converterFidelity');
      | blockPath = [gcb,'/','Converter','/',converterFidelity,'/','Converter'];
      | component.mask.openBlock(blockPath);
      mask Display: image('battery_1.png');
  Filter & Measurements : Subsystem
  ~ : PMIOPort  Side=Right
  Meas : Outport
  wires:
  BESS Plant/1(SOC) -> Filter & Measurements/1(SOC)
  FRef/1 -> BESS Controller/2(FRef)
  Mode/1 -> BESS Controller/5(Mode)
  PRef/1 -> BESS Controller/3(PRef)
  Filter & Measurements/1(VIBus) -> BESS Controller/7(VIBus)
  QRef/1 -> BESS Controller/4(QRef)
  VRef/1 -> BESS Controller/1(VRef)
  Reset/1 -> BESS Controller/6(Reset)
  Filter & Measurements/2(Meas) -> Meas/1
  BESS Controller/1(mabc) -> BESS Plant/1(mabc)
  connections:
  Filter & Measurements/RConn1 -- ~/RConn1
  BESS Plant/RConn1 -- Filter & Measurements/LConn1

== system MicrogridControl/BESS/BESS Integrated1/Simplified ==
  VRef : Inport
  FRef : Inport  Port=2
  PRef : Inport  Port=3
  QRef : Inport  Port=4
  Mode : Inport  Port=5
  Reset : Inport  Port=6
  Grid Following : Subsystem  VariantControl=Grid Following  mask(BESS GFL Simplified){plantRating=plantRating, Vac=Vac, frequency=frequency, iMaxPU=iMaxPU, efficiency=efficiency, bessVoltage=baseVoltageDC, maxSOC=maxSOC, minSOC=minSOC}
      mask prompts: plantRating "BESS Rating (kW)"; Vac "Rated AC side voltage (phase-phase RMS) (V)"; frequency "Rated electrical frequency at AC side (Hz)"; iMaxPU "Maximum converter current (pu)"; efficiency "Converter Efficiency (%)"; bessVoltage "Nominal BESS voltage (V)"; maxSOC "Maximum operating SOC"; minSOC "Minimum operating SOC"
      mask help: This block models a BESS that synchronizes with grid voltage and frequency using simplified control representation. This block is designed for computational efficiency, ideal for system-level studies in strong grid conditions where detailed transient behavior is less critical.
      settings: CopyFcn=set_param(gcbh,'LinkStatus','none');
      mask DialogControl generalDetailed Prompt: General
      mask DialogControl Container5 Prompt: Battery
      mask DialogControl editBattery Prompt: Edit battery parameters
      mask DialogControl editBattery Callback:
      | blockPath = [gcb,'/','Battery'] ;
      | component.mask.openBlock(blockPath);
  Grid Forming : Subsystem  VariantControl=Grid Forming  mask(BESS GFM Simplified){plantRating=plantRating, Vac=Vac, frequency=frequency, Vdc=baseVoltageDC, iMaxPU=iMaxPU, efficiency=efficiency, activeDroop=activeDroop, reactiveDroop=reactiveDroop, initialSOC=initialSOC, maxSOC=0.95, minSOC=0.1, capacityType=Infinite, capacity=capacity}
      mask prompts: plantRating "BESS Rating (kW)"; Vac "Rated AC side voltage (phase-phase RMS) (V)"; frequency "Rated electrical frequency at AC side (Hz)"; Vdc "Nominal DC bus voltage (V)"; iMaxPU "Maximum converter current (pu)"; efficiency "Converter Efficiency (%)"; activeDroop "Active droop"; reactiveDroop "Reactive droop"; initialSOC "Initial SOC"; maxSOC "Maximum operating SOC"; minSOC "Minimum operating SOC"; capacityType "Battery charge capacity"; capacity "Battery capacity (Ah)"
      mask help: This block models a BESS with generating voltage and frequency reference capabilities. It is optimized for faster simulations while maintaining essential grid-forming behavior, making it suitable for large-scale stability studies or planning scenarios where detailed converter dynamics are not required.
      settings: CopyFcn=set_param(gcbh,'LinkStatus','none');
      mask TypeOptions capacityType: Fixed | Infinite
      mask Callback capacityType: component.mask.configureBatteryCapacity;
      mask DialogControl generalDetailed Prompt: General
      mask DialogControl Container5 Prompt: Battery
  ~ : PMIOPort  Side=Right
  Meas : Outport

== system MicrogridControl/BESS/BESS Integrated3/Detailed ==
  note: Plant
  note: Controller
  VRef : Inport
  FRef : Inport  Port=2
  PRef : Inport  Port=3
  QRef : Inport  Port=4
  Mode : Inport  Port=5
  Reset : Inport  Port=6
  BESS Controller : Subsystem  Variant=on  VariantControlMode=label  LabelModeActiveChoice=Grid Forming
  BESS Plant : Subsystem  mask(BESS Plant){converterFidelity=Average, fSw=fSw, ratedVoltage=Vac}
      mask prompts: converterFidelity "Converter Fidelity"; fSw "Switching Frequency (kHz)"; ratedVoltage "Rated voltage on AC side (V)"
      mask help: This block represents the physical interface between the battery and the power converter. It models the electrical and dynamic characteristics of the battery system connected to a converter, while expecting an external control signal for operation
      settings: CopyFcn=set_param(gcbh,'LinkStatus','none');
      mask TypeOptions converterFidelity: Converter/converterFidelity
      mask Callback converterFidelity: component.mask.converterFidelityPlant;
      mask TypeOptions fSw: Converter/fSw
      mask DialogControl Container4 Prompt: General
      mask DialogControl editBattery Prompt: Edit battery parameters
      mask DialogControl editBattery Callback:
      | blockPath = [gcb,'/','Battery'];
      | component.mask.openBlock(blockPath);
      mask DialogControl editConverter Prompt: Edit converter parameters
      mask DialogControl editConverter Callback:
      | converterFidelity = get_param(gcb,'converterFidelity');
      | blockPath = [gcb,'/','Converter','/',converterFidelity,'/','Converter'];
      | component.mask.openBlock(blockPath);
      mask Display: image('battery_2.png');
  Filter & Measurements : Subsystem
  ~ : PMIOPort  Side=Right
  Meas : Outport
  wires:
  BESS Plant/1(SOC) -> Filter & Measurements/1(SOC)
  FRef/1 -> BESS Controller/2(FRef)
  Mode/1 -> BESS Controller/5(Mode)
  PRef/1 -> BESS Controller/3(PRef)
  Filter & Measurements/1(VIBus) -> BESS Controller/7(VIBus)
  QRef/1 -> BESS Controller/4(QRef)
  VRef/1 -> BESS Controller/1(VRef)
  Reset/1 -> BESS Controller/6(Reset)
  Filter & Measurements/2(Meas) -> Meas/1
  BESS Controller/1(mabc) -> BESS Plant/1(mabc)
  connections:
  Filter & Measurements/RConn1 -- ~/RConn1
  BESS Plant/RConn1 -- Filter & Measurements/LConn1

== system MicrogridControl/BESS/BESS Integrated3/Simplified ==
  VRef : Inport
  FRef : Inport  Port=2
  PRef : Inport  Port=3
  QRef : Inport  Port=4
  Mode : Inport  Port=5
  Reset : Inport  Port=6
  Grid Following : Subsystem  VariantControl=Grid Following  mask(BESS GFL Simplified){plantRating=plantRating, Vac=Vac, frequency=frequency, iMaxPU=iMaxPU, efficiency=efficiency, bessVoltage=baseVoltageDC, maxSOC=maxSOC, minSOC=minSOC}
      mask prompts: plantRating "BESS Rating (kW)"; Vac "Rated AC side voltage (phase-phase RMS) (V)"; frequency "Rated electrical frequency at AC side (Hz)"; iMaxPU "Maximum converter current (pu)"; efficiency "Converter Efficiency (%)"; bessVoltage "Nominal BESS voltage (V)"; maxSOC "Maximum operating SOC"; minSOC "Minimum operating SOC"
      mask help: This block models a BESS that synchronizes with grid voltage and frequency using simplified control representation. This block is designed for computational efficiency, ideal for system-level studies in strong grid conditions where detailed transient behavior is less critical.
      settings: CopyFcn=set_param(gcbh,'LinkStatus','none');
      mask DialogControl generalDetailed Prompt: General
      mask DialogControl Container5 Prompt: Battery
      mask DialogControl editBattery Prompt: Edit battery parameters
      mask DialogControl editBattery Callback:
      | blockPath = [gcb,'/','Battery'] ;
      | component.mask.openBlock(blockPath);
  Grid Forming : Subsystem  VariantControl=Grid Forming  mask(BESS GFM Simplified){plantRating=plantRating, Vac=Vac, frequency=frequency, Vdc=baseVoltageDC, iMaxPU=iMaxPU, efficiency=efficiency, activeDroop=activeDroop, reactiveDroop=reactiveDroop, initialSOC=initialSOC, maxSOC=0.95, minSOC=0.1, capacityType=Infinite, capacity=capacity}
      mask prompts: plantRating "BESS Rating (kW)"; Vac "Rated AC side voltage (phase-phase RMS) (V)"; frequency "Rated electrical frequency at AC side (Hz)"; Vdc "Nominal DC bus voltage (V)"; iMaxPU "Maximum converter current (pu)"; efficiency "Converter Efficiency (%)"; activeDroop "Active droop"; reactiveDroop "Reactive droop"; initialSOC "Initial SOC"; maxSOC "Maximum operating SOC"; minSOC "Minimum operating SOC"; capacityType "Battery charge capacity"; capacity "Battery capacity (Ah)"
      mask help: This block models a BESS with generating voltage and frequency reference capabilities. It is optimized for faster simulations while maintaining essential grid-forming behavior, making it suitable for large-scale stability studies or planning scenarios where detailed converter dynamics are not required.
      settings: CopyFcn=set_param(gcbh,'LinkStatus','none');
      mask TypeOptions capacityType: Fixed | Infinite
      mask Callback capacityType: component.mask.configureBatteryCapacity;
      mask DialogControl generalDetailed Prompt: General
      mask DialogControl Container5 Prompt: Battery
  ~ : PMIOPort  Side=Right
  Meas : Outport

== system MicrogridControl/BESS/Transformer/Detailed ==
  Two-Winding Transformer (Three-Phase)1 : ee_lib/Passive/Transformers/Two-Winding Transformer (Three-Phase)  SRated=3e6 A*V  FRated=systemFrequency Hz  Winding1Connection=ee.enum.windingconnection.Yg  VRated1=690 V  Winding2Connection=ee.enum.windingconnection.Yg  VRated2=11000 V  CoreType=ee.enum.coretype.threelimb  pu_Rw1=0.01  pu_Rw2=0.01  leakage_reactance_option=ee.enum.transformer_leakage.include  pu_Xl1=0.05  pu_Xl2=0.05  magnetizing_resistance_option=ee.enum.transformer_magnetizingResistance.include  pu_Rm=500  magnetizing_reactance_option=ee.enum.transformer_magnetizingReactance.include  saturation_option=ee.enum.transformer_saturation.exclude  pu_Xm=500  current_data=[0, .002, 1, 2]  magnetic_flux_data=[0, 1.2, 1.5, 1.51]  pu_X0=0.5  i1_specify=off  i1_priority=None  i1=[0, 0, 0] A  i1_nominal_specify=off  i1_nominal_value=1  i1_nominal_unit=A  i2_specify=off  i2_priority=None  i2=[0, 0, 0] A  i2_nominal_specify=off  i2_nominal_value=1  i2_nominal_unit=A  phi_specify=off  phi_priority=None  phi=[0, 0, 0]  phi_nominal_specify=off  phi_nominal_value=1  phi_nominal_unit=1  power_dissipated_specify=off  power_dissipated_priority=None  power_dissipated=0 W  power_dissipated_nominal_specify=off  power_dissipated_nominal_value=1  power_dissipated_nominal_unit=W
      settings: InternalSimscapePortConfiguration="{\"Bottom\":[],\"Left\":[{\"id\":\"N1\",\"label\":\"~1\",\"type\":\"foundation.electrical.three_phase\"}],\"Right\":[{\"id\":\"N2\",\"label\":\"~2\",\"type\":\"foundation.electrical.three_phase\"}],\"Top\":[]}"
  In : PMIOPort  Side=Left
  Out : PMIOPort  Port=2  Side=Right
  connections:
  Two-Winding Transformer (Three-Phase)1/LConn1 -- In/RConn1
  Two-Winding Transformer (Three-Phase)1/RConn1 -- Out/RConn1
